simulink model "fcaa"  (R2023a)
settings: Solver=VariableStepAuto  StartTime=0.0  StopTime=10.0  RelTol=1e-3
settings Model: Creator=ardasengenc  LastModifiedBy=ardasengenc

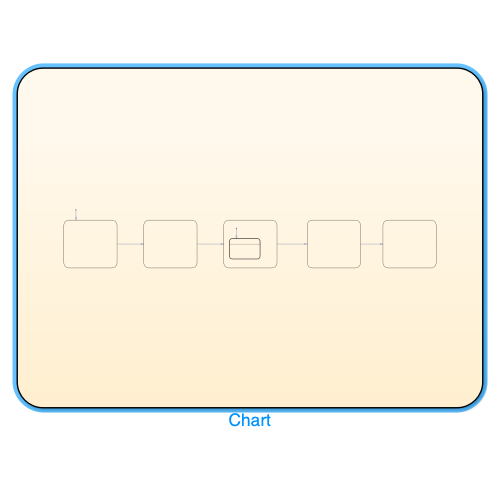
[thumbnail: Simulink's stored preview of the top-level diagram]
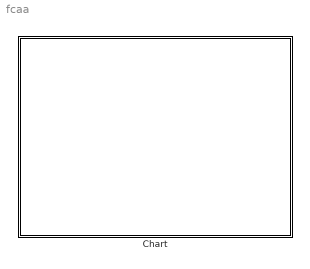
== system fcaa ==
  Chart : Stateflow chart  TreatAsAtomicUnit=on

== stateflow chart fcaa/Chart ==
  state Standby
  state Warning
  state Decision
    state DecisionTree
      state Start
      state Ignore
      state Brake
        state BrakeAlgo
      state Evasion
        state EvasionAlgorithm
          state DetermineAction
          state LeftLaneClear
          state RightLaneClear
          (default) -> DetermineAction
          DetermineAction -> LeftLaneClear [order 2]
          DetermineAction -> RightLaneClear [order 1]
      (default) -> Start
      Start -> Brake [order 1]
      Start -> Evasion [order 2]
      Start -> Ignore [order 3]
    (default) -> DecisionTree
  state Control
  state Completed
  (default) -> Standby
  Standby -> Warning
  Warning -> Decision
  Decision -> Control
  Control -> Completed
  Completed -> Standby
